simulink model "SpeedgoatCANOpen07"  (R2018b)
settings: Solver=FixedStepDiscrete  StartTime=0.0  StopTime=inf  FixedStep=0.0001  RelTol=1e-3  EnableMultiTasking=on
libraries: slrtlib x9, speedgoatlib_IO691 x5
(part 2 of 2)

== stateflow chart SpeedgoatCANOpen07/Trike Application Layer/Set_0_pos_homing1 ==
  state Init
    entry:
    % control word
    x1r        = 0;         % reset
    x2r        = 128;     % reset error
    x1_cw   = 6;         % shutdown
    x2_cw   = 7;         % switchon
    x3_cw   = 15;       % operationenable
    x4_cw   = 31;       % start homing / set 0 point
    % status word
    x1r2r_sw = 576;
    x1_sw = 545;     % status for shutdown
    x2_sw = 563;     % status for switchon
    x3_sw = 1591;   % status for operationenable
    x4_sw = 5687;   % status for homing / set 0 point
    aux=0;
    aux2=0;
    %OpMode = 1;
  state Not_assume_target_pos
    du:
    ControlWord = 15;%79 x3_cw;   2F
    aux2 = aux2+1;
  state SetHomingMode
    du:
    OpMode = 6;
    enable=0;
    aux2=aux2+1;
  state ShutDown
    du:
    ControlWord = x1_cw;
    aux2=aux2+1;
  state SwitchOn
    du:
    ControlWord = x2_cw;
    aux2=aux2+1;
  state Set_target_position
    en:
    aux=aux+1000;
    du:
    TargetPosition=aux;
    aux2 = aux2+1;
  state Homing_Set0Pos
    du:
    ControlWord = x4_cw;
    aux2=aux2+1;
  state OperationEnable
    du:
    ControlWord = x3_cw;
    aux2=aux2+1;
  state OperationEnable1
    du:
    ControlWord = x3_cw;
    enable=1;
    aux2=aux2+1;
  state SetOpMode_PositionMode
    du:
    OpMode = 1;
    aux2=aux2+1;
  state Assume_target_pos
    du:
    ControlWord = 31; %95 x4_cw;  3F
    aux2 = aux2+1;
  state OperationEnable2
    du:
    ControlWord = x3_cw;
    aux2=aux2+1;
  (default) -> Init
  Init -> Not_assume_target_pos [order 2] : [StatusWord==x3_sw && enable==1]{after(1000,tick)}
  Assume_target_pos -> Not_assume_target_pos : [aux2>100]{after(1000,tick), aux2=0}
  Not_assume_target_pos -> Set_target_position : [aux2>100]{after(1000,tick), aux2=0}
  SetHomingMode -> ShutDown : [StatusOpMode==6 && aux2>1000]{after(1000,tick), aux2=0}
  ShutDown -> SwitchOn : [StatusWord==x1_sw && aux2>1000]{after(1000,tick), aux2=0}
  Init -> SetHomingMode [order 1] : [B7==1]
  OperationEnable1 -> Init : [StatusWord==x3_sw && StatusOpMode==1 && aux2>1000]{after(1000,tick), aux2=0}
  SwitchOn -> OperationEnable : [StatusWord==x2_sw && aux2>1000]{after(1000,tick), aux2=0}
  Set_target_position -> Assume_target_pos : [aux2>100]{after(1000,tick), aux2=0}
  SetOpMode_PositionMode -> OperationEnable1 : [StatusWord==x3_sw && StatusOpMode==1 && aux2>1000]{after(1000,tick), aux2=0}
  OperationEnable -> Homing_Set0Pos : [StatusWord==567 && aux2>1000]{after(1000,tick), aux2=0}
  Homing_Set0Pos -> OperationEnable2 : [StatusWord==x4_sw && aux2>1000]{after(1000,tick), aux2=0}
  OperationEnable2 -> SetOpMode_PositionMode : [StatusWord==x4_sw  && aux2>1000]{after(1000,tick), aux2=0}
  data: StatusWord input; PowerOn input; B7 input; ControlWord output; OpMode output; x1_cw local; x2_cw local; x3_cw local; x4_cw local; x1r local; x1_sw local; x2_sw local; x3_sw local; x4_sw local; x2r local; TargetPosition output; Target input; StatusOpMode input; x1r2r_sw local; aux2 local; oldPosition local; x5s1 local; aux local; enable local

== matlab function SpeedgoatCANOpen07/Trike Application Layer/MATLAB Function1 ==
  data: ButtonStatus input; B7 output
function B7 = Button7Check(ButtonStatus)
aux =1;
if (ButtonStatus==64)
        aux = 2;
else 
    aux =1;
 end
B7 =aux;

== stateflow chart SpeedgoatCANOpen07/Trike Application Layer/ElectricDrive_state_machine1 ==
  state Init
    entry:
    % control word
    x1   = 3;         % switchon_disabled
    x2   = 6;         % switchon_ready
    x3   = 7;         % switchon
    x4   = 15;       % operationenable
    x5   = 2;         % quiqstop
    % status word
    x1s = 576;     % status for switchon_disabled
    x3s = 563;     % status for switchon_ready
    x2s = 545;     % status for  switchon_ready
    x4s = 5687;   % status for operationenable
    x5s = 576;     % status for quiqstop
  state SwitchOn_Disabled
    entry:
    ControlWord=x1;
  state SwitchOn_Ready
    entry:
    ControlWord=x2;
  state SwitchOn
    entry:
    ControlWord=x3;
  state QuiqStop
    entry:
    ControlWord=x5;
  state OperationEnable
    entry:
    ControlWord=x4;
  (default) -> Init
  SwitchOn_Disabled -> SwitchOn_Ready : [StatusWord==x1s && PowerOn==1]{after(10,tick)}
  SwitchOn_Ready -> SwitchOn [order 2] : [StatusWord==x2s && PowerOn==1]{after(10,tick)}
  SwitchOn_Ready -> SwitchOn_Disabled [order 1] : [StatusWord==x2s && PowerOn==0]{after(10,tick)}
  SwitchOn -> SwitchOn_Ready [order 1] : [StatusWord==x3s && PowerOn==0]{after(10,tick)}
  Init -> SwitchOn_Disabled
  QuiqStop -> SwitchOn_Disabled : [StatusWord==x5s && PowerOn==0]{after(10,tick)}
  OperationEnable -> SwitchOn [order 1] : [StatusWord==x4s && PowerOn==0]{after(10,tick)}
  SwitchOn -> OperationEnable [order 2] : [StatusWord==x3s && PowerOn==1]{after(10,tick)}
  OperationEnable -> QuiqStop [order 2] : [StatusWord==x4s && PowerOn==0]{after(10,tick)}
  data: StatusWord input; PowerOn input; ControlWord output; x1 local; x2 local; x3 local; x4 local; x5 local; x1s local; x2s local; x3s local; x4s local; x5s local

== matlab function SpeedgoatCANOpen07/Trike Application Layer/MATLAB Function4 ==
  data: ButtonStatus input; Byte0 output
function Byte0 = PowerOn(ButtonStatus)
Power =0;
if (ButtonStatus>=127)
        Power = 1;
else 
    Power =0;
 end
Byte0 =Power;

== stateflow chart SpeedgoatCANOpen07/Trike Application Layer/Set_0_pos_homing ==
  state Init
    entry:
    % control word
    x1r        = 0;         % reset
    x2r        = 128;     % reset error
    x1_cw   = 6;         % shutdown
    x2_cw   = 7;         % switchon
    x3_cw   = 15;       % operationenable
    x4_cw   = 31;       % start homing / set 0 point
    % status word
    x1r2r_sw = 576;
    x1_sw = 545;     % status for shutdown
    x2_sw = 563;     % status for switchon
    x3_sw = 1591;   % status for operationenable
    x4_sw = 5687;   % status for homing / set 0 point
    aux=0;
    aux2=0;
    %OpMode = 1;
  state Not_assume_target_pos
    du:
    ControlWord = 15;%79 x3_cw;   2F
    aux2 = aux2+1;
  state SetHomingMode
    du:
    OpMode = 6;
    enable=0;
    aux2=aux2+1;
  state ShutDown
    du:
    ControlWord = x1_cw;
    aux2=aux2+1;
  state SwitchOn
    du:
    ControlWord = x2_cw;
    aux2=aux2+1;
  state Set_target_position
    en:
    aux=aux+2000;
    du:
    TargetPosition=Target;
    aux2 = aux2+1;
  state Homing_Set0Pos
    du:
    ControlWord = x4_cw;
    aux2=aux2+1;
  state OperationEnable
    du:
    ControlWord = x3_cw;
    aux2=aux2+1;
  state OperationEnable1
    du:
    ControlWord = x3_cw;
    enable=1;
    aux2=aux2+1;
  state SetOpMode_PositionMode
    du:
    OpMode = 1;
    aux2=aux2+1;
  state Assume_target_pos
    du:
    ControlWord = 31; %95 x4_cw;  3F
    aux2 = aux2+1;
  state OperationEnable2
    du:
    ControlWord = x3_cw;
    aux2=aux2+1;
  (default) -> Init
  Init -> Not_assume_target_pos [order 2] : [StatusWord==x3_sw && enable==1]{after(1000,tick)}
  Assume_target_pos -> Not_assume_target_pos : [StatusWord==x4_sw ||  StatusWord==4663]{after(10,tick), aux2=0}
  Not_assume_target_pos -> Set_target_position : [StatusWord==x3_sw ]{after(10,tick), aux2=0}
  SetHomingMode -> ShutDown : [StatusOpMode==6 && aux2>1000]{after(1000,tick), aux2=0}
  ShutDown -> SwitchOn : [StatusWord==x1_sw && aux2>1000]{after(1000,tick), aux2=0}
  Init -> SetHomingMode [order 1] : [B7==1]
  OperationEnable1 -> Init : [StatusWord==x3_sw && StatusOpMode==1 && aux2>1000]{after(1000,tick), aux2=0}
  SwitchOn -> OperationEnable : [StatusWord==x2_sw && aux2>1000]{after(1000,tick), aux2=0}
  Set_target_position -> Assume_target_pos : [aux2>1]{after(10,tick), aux2=0}
  SetOpMode_PositionMode -> OperationEnable1 : [StatusWord==x3_sw && StatusOpMode==1 && aux2>1000]{after(1000,tick), aux2=0}
  OperationEnable -> Homing_Set0Pos : [StatusWord==567 && aux2>1000]{after(1000,tick), aux2=0}
  Homing_Set0Pos -> OperationEnable2 : [StatusWord==x4_sw && aux2>1000]{after(1000,tick), aux2=0}
  OperationEnable2 -> SetOpMode_PositionMode : [StatusWord==x4_sw  && aux2>1000]{after(1000,tick), aux2=0}
  data: StatusWord input; PowerOn input; B7 input; ControlWord output; OpMode output; x1_cw local; x2_cw local; x3_cw local; x4_cw local; x1r local; x1_sw local; x2_sw local; x3_sw local; x4_sw local; x2r local; TargetPosition output; Target input; StatusOpMode input; x1r2r_sw local; aux2 local; oldPosition local; x5s1 local; aux local; enable local

== matlab function SpeedgoatCANOpen07/Trike Application Layer/MATLAB Function6 ==
  data: ButtonStatus input; B8 output
function B8 = PowerOn(ButtonStatus)
Power =0;
if (ButtonStatus>=127)
        Power = 1;
else 
    Power =0;
 end
B8 =Power;

== matlab function SpeedgoatCANOpen07/Trike Application Layer/MATLAB Function7 ==
  data: ButtonStatus input; B7 output
function B7 = Button7Check(ButtonStatus)
aux =0;
if (ButtonStatus==64)
        aux =1;
else 
    aux =0;
 end
B7 =aux;
